simulink model "fmudemo_vdp"  (R2022b)
settings: Solver=VariableStepAuto  StartTime=0.0  StopTime=10.0  RelTol=1e-3
model workspace (MAT data in the model file):
  Flow = Simulink.Parameter
  Flow.DataType = 'double'
  Flow.Complexity = 'real'
  Flow.Dimensions = [0 0]
Description:
  | Importing a Co-Simulation FMU into Simulink
  | 
  | This model shows how to use the FMU Import block to load an FMU file. The FMU file supports execution in Co-Simulation mode.
settings Model: Creator=The MathWorks, Inc.  LastModifiedBy=anna.reale
settings SolverCC: AlgebraicLoopSolver=TrustRegion
settings DebuggingCC: UnconnectedInputMsg=warning  UnconnectedOutputMsg=warning  UnconnectedLineMsg=warning  SFMachineParentedDataDiag=warning  ArithmeticOperatorsInVariantConditions=warning
settings ModelReferenceCC: EnableRefExpFcnMdlSchedulingChecks=on
settings SFSimCC: SimUseLocalCustomCode=off  CustomCodeUndefinedFunction=UseInterfaceOnly
settings RTWCC: RTWUseLocalCustomCode=off  DLArmComputeVersion=19.05

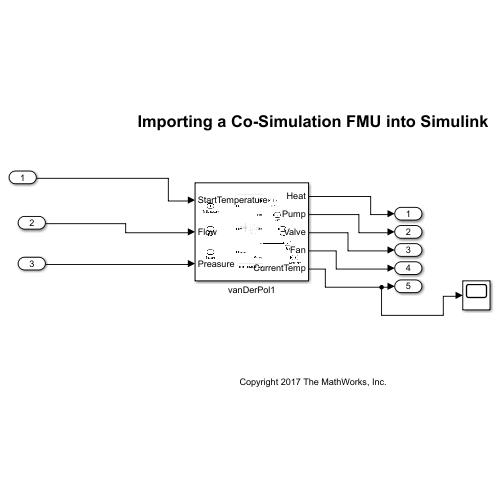
[thumbnail: Simulink's stored preview of the top-level diagram]
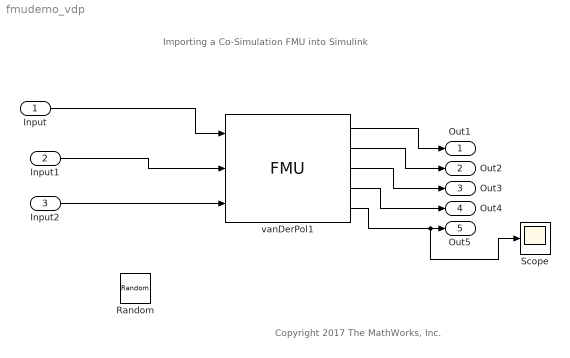
== system fmudemo_vdp ==
  note: Copyright 2017 The MathWorks, Inc.
  note: Importing a Co-Simulation FMU into Simulink
  Input : Inport  OutDataTypeStr=double
  Input1 : Inport  Port=2  OutDataTypeStr=double
  Input2 : Inport  Port=3  OutDataTypeStr=double
  Scope : Scope
  vanDerPol1 : FMU  FMUName=TMS_FMU_Hackathon_Input.fmu  FMUMode=CoSimulation  FMUSampleTime=0.1  FMUCreateBusObject=off
      mask Type: FMUControllerLogicSingleHackathon [Co-Simulation, v2.0]
      mask Display:
      | if (exist([Simulink.fileGenControl('get','CacheFolder') '\slprj\_fmu\e25485790cc2c8632848a33da27c9699\TMS_FMU_Hackathon_Input\model.png'],'file'))
      |     image([Simulink.fileGenControl('get','CacheFolder') '\slprj\_fmu\e25485790cc2c8632848a33da27c9699\TMS_FMU_Hackathon_Input\model.png']);
      | else
      |     disp('FMUControllerLogicSingleHackathon');
      | end
      | port_label('output',1,'Heat');
      | port_label('output',2,'Pump');
      | port_label('output',3,'Valve');
      | port_label('output',4,'Fan');
      | port_label('output',5,'CurrentTemp');
      | port_label('input',1,'StartTemperature');
      | port_label('input',2,'Flow');
      | port_label('input',3,'Preasure');
  Out1 : Outport
  Out2 : Outport  Port=2
  Out3 : Outport  Port=3
  Out4 : Outport  Port=4
  Out5 : Outport  Port=5
  Random : RandomNumber  IOType=siggen  SampleTime=0
  wires:
  vanDerPol1/1 -> Out1/1
  vanDerPol1/2 -> Out2/1
  vanDerPol1/3 -> Out3/1
  vanDerPol1/4 -> Out4/1
  vanDerPol1/5 -> Scope/1, Out5/1
  Input/1 -> vanDerPol1/1
  Input1/1 -> vanDerPol1/2
  Input2/1 -> vanDerPol1/3
